simulink model "CMOS_Kernel_Memory_Sync"  (R2023b)
settings: Solver=VariableStepAuto  StartTime=0.0  StopTime=30000000  RelTol=1e-3
values from neighbouring files (symbols this model uses):
  AmountOfPixelsPerScanline = 400    [Kernel_Setup_Script.m]
  AmountOfRamBlocksScanlines = 5    [Kernel_Setup_Script.m]
  AmountOfRamBlocksScanlinesOffset = AmountOfRamBlocksScanlines - 1    (= 4)    [Kernel_Setup_Script.m]
  AmountOfScanlinePixels = 73700    [Kernel_Setup_Script.m]
  AmountOfScanlinePixelsOffset = AmountOfScanlinePixels - 1    (= 73699)    [Kernel_Setup_Script.m]
  AmountOfScanlines = 1100    [Kernel_Setup_Script.m]
  AmountOfScanlinesOffset = AmountOfScanlines - 1    (= 1099)    [Kernel_Setup_Script.m]
  AOPPK_Off = AmountOfPixelsPerScanline - 1    (= 399)    [Kernel_Setup_Script.m]
  AOPPS_Off = AmountOfPixelsPerScanline - 1    (= 399)    [Kernel_Setup_Script.m]
  FramePackOff_0 = FramePackOff_0 - ScanlineFifoCheck    [Kernel_Setup_Script.m]
  FramePackOff_1 = FramePackOff_1 - ScanlineFifoCheck    [Kernel_Setup_Script.m]
  FramePackOff_2 = FramePackOff_2 - ScanlineFifoCheck    [Kernel_Setup_Script.m]
  FramePackOff_3 = FramePackOff_3 - ScanlineFifoCheck    [Kernel_Setup_Script.m]
  FramePackOff_4 = FramePackOff_4 - ScanlineFifoCheck    [Kernel_Setup_Script.m]
  FramePackOff_5 = FramePackOff_5 - ScanlineFifoCheck    [Kernel_Setup_Script.m]
  KernelPackOff_0 = KernelPackOff_0 - KernelBitsPerRow    [Kernel_Setup_Script.m]
  KernelPackOff_1 = KernelPackOff_1 - KernelBitsPerRow    [Kernel_Setup_Script.m]
  KernelPackOff_2 = KernelPackOff_2 - KernelBitsPerRow    [Kernel_Setup_Script.m]
  KernelPackOff_3 = KernelPackOff_3 - KernelBitsPerRow    [Kernel_Setup_Script.m]
  Slice59DownTo48Top = (MsbOffset - (ScanlinePixelBitSizeController*1))    (= 59)    [Kernel_Setup_Script.m]
  Slice71DownTo60Top = (MsbOffset - (ScanlinePixelBitSizeController*0))    (= 71)    [Kernel_Setup_Script.m]
  TotalSectionsForFrames = AmountOfScanlines/AmountOfRamBlocksScanlines    (= 220)    [Kernel_Setup_Script.m]
  UltraRamRows = AmountOfPixelsPerScanline/ScanlineFifoCheck    [Kernel_Setup_Script.m]
  UltraRamRowsCeil = ceil(AmountOfPixelsPerScanline/ScanlineFifoCheck)    [Kernel_Setup_Script.m]
  UltraRamRowsKernel = AmountOfPixelsPerScanline/KernelBitsPerRow    (= 100)    [Kernel_Setup_Script.m]
  UltraRamRowsKernelCeil = ceil(AmountOfPixelsPerScanline/KernelBitsPerRow)    [Kernel_Setup_Script.m]
  UltraRamRowsMemorySectionOffset = UltraRamRowsCeil*AmountOfRamBlocksScanlines    [Kernel_Setup_Script.m]
  UltraRamRowsOffset = UltraRamRowsCeil - 1    [Kernel_Setup_Script.m]
undefined symbols (not defined in the file or in its folder): c, Down, sfvc784, Up, xck26
libraries: hdlBasic x4512, vmcUtilities x1
(part 37 of 39)

== system CMOS_Kernel_Memory_Sync/Memory Handler/Memory Manager/Kernel Memory Subsystem/RAM Selector 2 ==
  Data In : Inport
  RAM Select : Inport  Port=2
  Constant1 : hdlBasic/Constant  const=0  gui_display_data_type=Boolean  arith_type=Boolean  n_bits=1  bin_pt=0  preci_type=Single  exp_width=8  frac_width=24  explicit_period=off  period=1  XmcBlockStatus=1  maskContainerNames=tabcontainer1  block_type=constant  block_config=sysgen:Constant_config
  Delay : hdlBasic/Delay  rst=off  en=off  latency=1  reg_retiming=off  XmcBlockStatus=1  maskContainerNames=group1  block_type=delay  block_config=sysgen:Delay_config
  Line Out RAM {0..4} (5 alike) : hdlBasic/Mux  inputs=2  en=off  latency=1  precision=Full  arith_type=Unsigned  n_bits=16  bin_pt=14  quantization=Truncate  overflow=Wrap  XmcBlockStatus=1  maskContainerNames=tabcontainer1  block_type=mux  block_config=sysgen:Mux_config
  Sel RAM {0..4} (5 alike) : hdlBasic/Relational  mode=a=b  op_type=Bool  en=off  latency=1  XmcBlockStatus=1  maskContainerNames=tabcontainer1  block_type=relational  block_config=sysgen:Relational_config
  Sel Value RAM 0 : hdlBasic/Constant  const=0  gui_display_data_type=Fixed-point  arith_type=Unsigned  n_bits=3  bin_pt=0  preci_type=Single  exp_width=8  frac_width=24  explicit_period=off  period=1  XmcBlockStatus=1  maskContainerNames=tabcontainer1  block_type=constant  block_config=sysgen:Constant_config
  Sel Value RAM 1 : hdlBasic/Constant  const=1  gui_display_data_type=Fixed-point  arith_type=Unsigned  n_bits=3  bin_pt=0  preci_type=Single  exp_width=8  frac_width=24  explicit_period=off  period=1  XmcBlockStatus=1  maskContainerNames=tabcontainer1  block_type=constant  block_config=sysgen:Constant_config
  Sel Value RAM 2 : hdlBasic/Constant  const=2  gui_display_data_type=Fixed-point  arith_type=Unsigned  n_bits=3  bin_pt=0  preci_type=Single  exp_width=8  frac_width=24  explicit_period=off  period=1  XmcBlockStatus=1  maskContainerNames=tabcontainer1  block_type=constant  block_config=sysgen:Constant_config
  Sel Value RAM 3 : hdlBasic/Constant  const=3  gui_display_data_type=Fixed-point  arith_type=Unsigned  n_bits=3  bin_pt=0  preci_type=Single  exp_width=8  frac_width=24  explicit_period=off  period=1  XmcBlockStatus=1  maskContainerNames=tabcontainer1  block_type=constant  block_config=sysgen:Constant_config
  Sel Value RAM 4 : hdlBasic/Constant  const=4  gui_display_data_type=Fixed-point  arith_type=Unsigned  n_bits=3  bin_pt=0  preci_type=Single  exp_width=8  frac_width=24  explicit_period=off  period=1  XmcBlockStatus=1  maskContainerNames=tabcontainer1  block_type=constant  block_config=sysgen:Constant_config
  Out RAM 0 : Outport
  Out RAM 1 : Outport  Port=2
  Out RAM 2 : Outport  Port=3
  Out RAM 3 : Outport  Port=4
  Out RAM 4 : Outport  Port=5
  wires:
  Sel Value RAM 0/1 -> Sel RAM 0/2
  Sel Value RAM 1/1 -> Sel RAM 1/2
  Sel Value RAM 2/1 -> Sel RAM 2/2
  Sel Value RAM 3/1 -> Sel RAM 3/2
  Sel Value RAM 4/1 -> Sel RAM 4/2
  Delay/1 -> Line Out RAM 0/3, Line Out RAM 1/3, Line Out RAM 2/3, Line Out RAM 4/3, Line Out RAM 3/3
  Data In/1 -> Delay/1
  RAM Select/1 -> Sel RAM 4/1, Sel RAM 3/1, Sel RAM 2/1, Sel RAM 1/1, Sel RAM 0/1
  Line Out RAM 0/1 -> Out RAM 0/1
  Line Out RAM 1/1 -> Out RAM 1/1
  Line Out RAM 2/1 -> Out RAM 2/1
  Line Out RAM 3/1 -> Out RAM 3/1
  Line Out RAM 4/1 -> Out RAM 4/1
  Constant1/1 -> Line Out RAM 0/2, Line Out RAM 4/2, Line Out RAM 3/2, Line Out RAM 2/2, Line Out RAM 1/2
  Sel RAM 0/1 -> Line Out RAM 0/1
  Sel RAM 1/1 -> Line Out RAM 1/1
  Sel RAM 2/1 -> Line Out RAM 2/1
  Sel RAM 3/1 -> Line Out RAM 3/1
  Sel RAM 4/1 -> Line Out RAM 4/1

== system CMOS_Kernel_Memory_Sync/Memory Handler/Memory Manager/Scanline Memory Subsystem/RAM Selector 0 ==
  Data In : Inport
  RAM Select : Inport  Port=2
  Constant1 : hdlBasic/Constant  const=0  gui_display_data_type=Fixed-point  arith_type=Unsigned  n_bits=1  bin_pt=0  preci_type=Single  exp_width=8  frac_width=24  explicit_period=off  period=1  XmcBlockStatus=1  maskContainerNames=tabcontainer1  block_type=constant  block_config=sysgen:Constant_config
  Delay : hdlBasic/Delay  rst=off  en=off  latency=1  reg_retiming=off  XmcBlockStatus=1  maskContainerNames=group1  block_type=delay  block_config=sysgen:Delay_config
  Line Out RAM {0..4} (5 alike) : hdlBasic/Mux  inputs=2  en=off  latency=1  precision=Full  arith_type=Unsigned  n_bits=16  bin_pt=14  quantization=Truncate  overflow=Wrap  XmcBlockStatus=1  maskContainerNames=tabcontainer1  block_type=mux  block_config=sysgen:Mux_config
  Sel RAM {0..4} (5 alike) : hdlBasic/Relational  mode=a=b  op_type=Bool  en=off  latency=1  XmcBlockStatus=1  maskContainerNames=tabcontainer1  block_type=relational  block_config=sysgen:Relational_config
  Sel Value RAM 0 : hdlBasic/Constant  const=0  gui_display_data_type=Fixed-point  arith_type=Unsigned  n_bits=3  bin_pt=0  preci_type=Single  exp_width=8  frac_width=24  explicit_period=off  period=1  XmcBlockStatus=1  maskContainerNames=tabcontainer1  block_type=constant  block_config=sysgen:Constant_config
  Sel Value RAM 1 : hdlBasic/Constant  const=1  gui_display_data_type=Fixed-point  arith_type=Unsigned  n_bits=3  bin_pt=0  preci_type=Single  exp_width=8  frac_width=24  explicit_period=off  period=1  XmcBlockStatus=1  maskContainerNames=tabcontainer1  block_type=constant  block_config=sysgen:Constant_config
  Sel Value RAM 2 : hdlBasic/Constant  const=2  gui_display_data_type=Fixed-point  arith_type=Unsigned  n_bits=3  bin_pt=0  preci_type=Single  exp_width=8  frac_width=24  explicit_period=off  period=1  XmcBlockStatus=1  maskContainerNames=tabcontainer1  block_type=constant  block_config=sysgen:Constant_config
  Sel Value RAM 3 : hdlBasic/Constant  const=3  gui_display_data_type=Fixed-point  arith_type=Unsigned  n_bits=3  bin_pt=0  preci_type=Single  exp_width=8  frac_width=24  explicit_period=off  period=1  XmcBlockStatus=1  maskContainerNames=tabcontainer1  block_type=constant  block_config=sysgen:Constant_config
  Sel Value RAM 4 : hdlBasic/Constant  const=4  gui_display_data_type=Fixed-point  arith_type=Unsigned  n_bits=3  bin_pt=0  preci_type=Single  exp_width=8  frac_width=24  explicit_period=off  period=1  XmcBlockStatus=1  maskContainerNames=tabcontainer1  block_type=constant  block_config=sysgen:Constant_config
  Out RAM 0 : Outport
  Out RAM 1 : Outport  Port=2
  Out RAM 2 : Outport  Port=3
  Out RAM 3 : Outport  Port=4
  Out RAM 4 : Outport  Port=5
  wires:
  Sel Value RAM 0/1 -> Sel RAM 0/2
  Sel Value RAM 1/1 -> Sel RAM 1/2
  Sel Value RAM 2/1 -> Sel RAM 2/2
  Sel Value RAM 3/1 -> Sel RAM 3/2
  Sel Value RAM 4/1 -> Sel RAM 4/2
  Delay/1 -> Line Out RAM 0/3, Line Out RAM 1/3, Line Out RAM 2/3, Line Out RAM 4/3, Line Out RAM 3/3
  Data In/1 -> Delay/1
  RAM Select/1 -> Sel RAM 4/1, Sel RAM 3/1, Sel RAM 2/1, Sel RAM 1/1, Sel RAM 0/1
  Line Out RAM 0/1 -> Out RAM 0/1
  Line Out RAM 1/1 -> Out RAM 1/1
  Line Out RAM 2/1 -> Out RAM 2/1
  Line Out RAM 3/1 -> Out RAM 3/1
  Line Out RAM 4/1 -> Out RAM 4/1
  Constant1/1 -> Line Out RAM 0/2, Line Out RAM 4/2, Line Out RAM 3/2, Line Out RAM 2/2, Line Out RAM 1/2
  Sel RAM 0/1 -> Line Out RAM 0/1
  Sel RAM 1/1 -> Line Out RAM 1/1
  Sel RAM 2/1 -> Line Out RAM 2/1
  Sel RAM 3/1 -> Line Out RAM 3/1
  Sel RAM 4/1 -> Line Out RAM 4/1

== system CMOS_Kernel_Memory_Sync/Memory Handler/Memory Manager/Scanline Memory Subsystem/RAM Selector 1 ==
  Data In : Inport
  RAM Select : Inport  Port=2
  Constant1 : hdlBasic/Constant  const=0  gui_display_data_type=Fixed-point  arith_type=Unsigned  n_bits=1  bin_pt=0  preci_type=Single  exp_width=8  frac_width=24  explicit_period=off  period=1  XmcBlockStatus=1  maskContainerNames=tabcontainer1  block_type=constant  block_config=sysgen:Constant_config
  Delay : hdlBasic/Delay  rst=off  en=off  latency=1  reg_retiming=off  XmcBlockStatus=1  maskContainerNames=group1  block_type=delay  block_config=sysgen:Delay_config
  Line Out RAM {0..4} (5 alike) : hdlBasic/Mux  inputs=2  en=off  latency=1  precision=Full  arith_type=Unsigned  n_bits=16  bin_pt=14  quantization=Truncate  overflow=Wrap  XmcBlockStatus=1  maskContainerNames=tabcontainer1  block_type=mux  block_config=sysgen:Mux_config
  Sel RAM {0..4} (5 alike) : hdlBasic/Relational  mode=a=b  op_type=Bool  en=off  latency=1  XmcBlockStatus=1  maskContainerNames=tabcontainer1  block_type=relational  block_config=sysgen:Relational_config
  Sel Value RAM 0 : hdlBasic/Constant  const=0  gui_display_data_type=Fixed-point  arith_type=Unsigned  n_bits=3  bin_pt=0  preci_type=Single  exp_width=8  frac_width=24  explicit_period=off  period=1  XmcBlockStatus=1  maskContainerNames=tabcontainer1  block_type=constant  block_config=sysgen:Constant_config
  Sel Value RAM 1 : hdlBasic/Constant  const=1  gui_display_data_type=Fixed-point  arith_type=Unsigned  n_bits=3  bin_pt=0  preci_type=Single  exp_width=8  frac_width=24  explicit_period=off  period=1  XmcBlockStatus=1  maskContainerNames=tabcontainer1  block_type=constant  block_config=sysgen:Constant_config
  Sel Value RAM 2 : hdlBasic/Constant  const=2  gui_display_data_type=Fixed-point  arith_type=Unsigned  n_bits=3  bin_pt=0  preci_type=Single  exp_width=8  frac_width=24  explicit_period=off  period=1  XmcBlockStatus=1  maskContainerNames=tabcontainer1  block_type=constant  block_config=sysgen:Constant_config
  Sel Value RAM 3 : hdlBasic/Constant  const=3  gui_display_data_type=Fixed-point  arith_type=Unsigned  n_bits=3  bin_pt=0  preci_type=Single  exp_width=8  frac_width=24  explicit_period=off  period=1  XmcBlockStatus=1  maskContainerNames=tabcontainer1  block_type=constant  block_config=sysgen:Constant_config
  Sel Value RAM 4 : hdlBasic/Constant  const=4  gui_display_data_type=Fixed-point  arith_type=Unsigned  n_bits=3  bin_pt=0  preci_type=Single  exp_width=8  frac_width=24  explicit_period=off  period=1  XmcBlockStatus=1  maskContainerNames=tabcontainer1  block_type=constant  block_config=sysgen:Constant_config
  Out RAM 0 : Outport
  Out RAM 1 : Outport  Port=2
  Out RAM 2 : Outport  Port=3
  Out RAM 3 : Outport  Port=4
  Out RAM 4 : Outport  Port=5
  wires:
  Sel Value RAM 0/1 -> Sel RAM 0/2
  Sel Value RAM 1/1 -> Sel RAM 1/2
  Sel Value RAM 2/1 -> Sel RAM 2/2
  Sel Value RAM 3/1 -> Sel RAM 3/2
  Sel Value RAM 4/1 -> Sel RAM 4/2
  Delay/1 -> Line Out RAM 0/3, Line Out RAM 1/3, Line Out RAM 2/3, Line Out RAM 4/3, Line Out RAM 3/3
  Data In/1 -> Delay/1
  RAM Select/1 -> Sel RAM 4/1, Sel RAM 3/1, Sel RAM 2/1, Sel RAM 1/1, Sel RAM 0/1
  Line Out RAM 0/1 -> Out RAM 0/1
  Line Out RAM 1/1 -> Out RAM 1/1
  Line Out RAM 2/1 -> Out RAM 2/1
  Line Out RAM 3/1 -> Out RAM 3/1
  Line Out RAM 4/1 -> Out RAM 4/1
  Constant1/1 -> Line Out RAM 0/2, Line Out RAM 4/2, Line Out RAM 3/2, Line Out RAM 2/2, Line Out RAM 1/2
  Sel RAM 0/1 -> Line Out RAM 0/1
  Sel RAM 1/1 -> Line Out RAM 1/1
  Sel RAM 2/1 -> Line Out RAM 2/1
  Sel RAM 3/1 -> Line Out RAM 3/1
  Sel RAM 4/1 -> Line Out RAM 4/1

== system CMOS_Kernel_Memory_Sync/Memory Handler/Memory Manager/Scanline Memory Subsystem/RAM Selector 2 ==
  Data In : Inport
  RAM Select : Inport  Port=2
  Constant1 : hdlBasic/Constant  const=0  gui_display_data_type=Boolean  arith_type=Boolean  n_bits=1  bin_pt=0  preci_type=Single  exp_width=8  frac_width=24  explicit_period=off  period=1  XmcBlockStatus=1  maskContainerNames=tabcontainer1  block_type=constant  block_config=sysgen:Constant_config
  Delay : hdlBasic/Delay  rst=off  en=off  latency=1  reg_retiming=off  XmcBlockStatus=1  maskContainerNames=group1  block_type=delay  block_config=sysgen:Delay_config
  Line Out RAM {0..4} (5 alike) : hdlBasic/Mux  inputs=2  en=off  latency=1  precision=Full  arith_type=Unsigned  n_bits=16  bin_pt=14  quantization=Truncate  overflow=Wrap  XmcBlockStatus=1  maskContainerNames=tabcontainer1  block_type=mux  block_config=sysgen:Mux_config
  Sel RAM {0..4} (5 alike) : hdlBasic/Relational  mode=a=b  op_type=Bool  en=off  latency=1  XmcBlockStatus=1  maskContainerNames=tabcontainer1  block_type=relational  block_config=sysgen:Relational_config
  Sel Value RAM 0 : hdlBasic/Constant  const=0  gui_display_data_type=Fixed-point  arith_type=Unsigned  n_bits=3  bin_pt=0  preci_type=Single  exp_width=8  frac_width=24  explicit_period=off  period=1  XmcBlockStatus=1  maskContainerNames=tabcontainer1  block_type=constant  block_config=sysgen:Constant_config
  Sel Value RAM 1 : hdlBasic/Constant  const=1  gui_display_data_type=Fixed-point  arith_type=Unsigned  n_bits=3  bin_pt=0  preci_type=Single  exp_width=8  frac_width=24  explicit_period=off  period=1  XmcBlockStatus=1  maskContainerNames=tabcontainer1  block_type=constant  block_config=sysgen:Constant_config
  Sel Value RAM 2 : hdlBasic/Constant  const=2  gui_display_data_type=Fixed-point  arith_type=Unsigned  n_bits=3  bin_pt=0  preci_type=Single  exp_width=8  frac_width=24  explicit_period=off  period=1  XmcBlockStatus=1  maskContainerNames=tabcontainer1  block_type=constant  block_config=sysgen:Constant_config
  Sel Value RAM 3 : hdlBasic/Constant  const=3  gui_display_data_type=Fixed-point  arith_type=Unsigned  n_bits=3  bin_pt=0  preci_type=Single  exp_width=8  frac_width=24  explicit_period=off  period=1  XmcBlockStatus=1  maskContainerNames=tabcontainer1  block_type=constant  block_config=sysgen:Constant_config
  Sel Value RAM 4 : hdlBasic/Constant  const=4  gui_display_data_type=Fixed-point  arith_type=Unsigned  n_bits=3  bin_pt=0  preci_type=Single  exp_width=8  frac_width=24  explicit_period=off  period=1  XmcBlockStatus=1  maskContainerNames=tabcontainer1  block_type=constant  block_config=sysgen:Constant_config
  Out RAM 0 : Outport
  Out RAM 1 : Outport  Port=2
  Out RAM 2 : Outport  Port=3
  Out RAM 3 : Outport  Port=4
  Out RAM 4 : Outport  Port=5
  wires:
  Sel Value RAM 0/1 -> Sel RAM 0/2
  Sel Value RAM 1/1 -> Sel RAM 1/2
  Sel Value RAM 2/1 -> Sel RAM 2/2
  Sel Value RAM 3/1 -> Sel RAM 3/2
  Sel Value RAM 4/1 -> Sel RAM 4/2
  Delay/1 -> Line Out RAM 0/3, Line Out RAM 1/3, Line Out RAM 2/3, Line Out RAM 4/3, Line Out RAM 3/3
  Data In/1 -> Delay/1
  RAM Select/1 -> Sel RAM 4/1, Sel RAM 3/1, Sel RAM 2/1, Sel RAM 1/1, Sel RAM 0/1
  Line Out RAM 0/1 -> Out RAM 0/1
  Line Out RAM 1/1 -> Out RAM 1/1
  Line Out RAM 2/1 -> Out RAM 2/1
  Line Out RAM 3/1 -> Out RAM 3/1
  Line Out RAM 4/1 -> Out RAM 4/1
  Constant1/1 -> Line Out RAM 0/2, Line Out RAM 4/2, Line Out RAM 3/2, Line Out RAM 2/2, Line Out RAM 1/2
  Sel RAM 0/1 -> Line Out RAM 0/1
  Sel RAM 1/1 -> Line Out RAM 1/1
  Sel RAM 2/1 -> Line Out RAM 2/1
  Sel RAM 3/1 -> Line Out RAM 3/1
  Sel RAM 4/1 -> Line Out RAM 4/1

== system CMOS_Kernel_Memory_Sync/Memory Handler/Data Slicer/Frame RAM Slicer/72 Bit Unpacker RAM 0/Unpack 72 Bit FIFO 0 ==
  72 Bit Input : Inport
  Slice 11 Down To 0 : hdlBasic/Slice  nbits=ScanlinePixelBitSizeController  boolean_output=off  mode=Upper Bit Location + Width  bit1=Slice11DownTo0Top  base1=LSB of Input  bit0=0  base0=Binary Point of Input  XmcBlockStatus=1  maskContainerNames=group1  block_type=slice  block_config=sysgen:Slice_config
  Slice 23 Down To 12 : hdlBasic/Slice  nbits=ScanlinePixelBitSizeController  boolean_output=off  mode=Upper Bit Location + Width  bit1=Slice23DownTo12Top  base1=LSB of Input  bit0=12  base0=Binary Point of Input  XmcBlockStatus=1  maskContainerNames=group1  block_type=slice  block_config=sysgen:Slice_config
  Slice 35 Down To 24 : hdlBasic/Slice  nbits=ScanlinePixelBitSizeController  boolean_output=off  mode=Upper Bit Location + Width  bit1=Slice35DownTo24Top  base1=LSB of Input  bit0=24  base0=Binary Point of Input  XmcBlockStatus=1  maskContainerNames=group1  block_type=slice  block_config=sysgen:Slice_config
  Slice 47 Down To 36 : hdlBasic/Slice  nbits=ScanlinePixelBitSizeController  boolean_output=off  mode=Upper Bit Location + Width  bit1=Slice47DownTo36Top  base1=LSB of Input  bit0=36  base0=Binary Point of Input  XmcBlockStatus=1  maskContainerNames=group1  block_type=slice  block_config=sysgen:Slice_config
  Slice 59 Down To 48 : hdlBasic/Slice  nbits=ScanlinePixelBitSizeController  boolean_output=off  mode=Upper Bit Location + Width  bit1=Slice59DownTo48Top  base1=LSB of Input  bit0=Slice59DownTo48Top - 11  base0=LSB of Input  XmcBlockStatus=1  maskContainerNames=group1  block_type=slice  block_config=sysgen:Slice_config
  Slice 71 Down To 60 : hdlBasic/Slice  nbits=ScanlinePixelBitSizeController  boolean_output=off  mode=Upper Bit Location + Width  bit1=Slice71DownTo60Top  base1=LSB of Input  bit0=Slice71DownTo60Top - 12  base0=LSB of Input  XmcBlockStatus=1  maskContainerNames=group1  block_type=slice  block_config=sysgen:Slice_config
  71 Downto 60 : Outport
  59 Downto 48 : Outport  Port=2
  47 Downto 36 : Outport  Port=3
  35 Downto 24 : Outport  Port=4
  23 Downto 12 : Outport  Port=5
  11 Downto 0 : Outport  Port=6
  wires:
  72 Bit Input/1 -> Slice 11 Down To 0/1, Slice 23 Down To 12/1, Slice 35 Down To 24/1, Slice 47 Down To 36/1, Slice 59 Down To 48/1, Slice 71 Down To 60/1
  Slice 23 Down To 12/1 -> 23 Downto 12/1
  Slice 47 Down To 36/1 -> 47 Downto 36/1
  Slice 59 Down To 48/1 -> 59 Downto 48/1
  Slice 35 Down To 24/1 -> 35 Downto 24/1
  Slice 71 Down To 60/1 -> 71 Downto 60/1
  Slice 11 Down To 0/1 -> 11 Downto 0/1

== system CMOS_Kernel_Memory_Sync/Memory Handler/Data Slicer/Frame RAM Slicer/72 Bit Unpacker RAM 0/Unpack 72 Bit FIFO 1 ==
  72 Bit Input : Inport
  Slice 11 Down To 0 : hdlBasic/Slice  nbits=ScanlinePixelBitSizeController  boolean_output=off  mode=Upper Bit Location + Width  bit1=Slice11DownTo0Top  base1=LSB of Input  bit0=0  base0=Binary Point of Input  XmcBlockStatus=1  maskContainerNames=group1  block_type=slice  block_config=sysgen:Slice_config
  Slice 23 Down To 12 : hdlBasic/Slice  nbits=ScanlinePixelBitSizeController  boolean_output=off  mode=Upper Bit Location + Width  bit1=Slice23DownTo12Top  base1=LSB of Input  bit0=12  base0=Binary Point of Input  XmcBlockStatus=1  maskContainerNames=group1  block_type=slice  block_config=sysgen:Slice_config
  Slice 35 Down To 24 : hdlBasic/Slice  nbits=ScanlinePixelBitSizeController  boolean_output=off  mode=Upper Bit Location + Width  bit1=Slice35DownTo24Top  base1=LSB of Input  bit0=24  base0=Binary Point of Input  XmcBlockStatus=1  maskContainerNames=group1  block_type=slice  block_config=sysgen:Slice_config
  Slice 47 Down To 36 : hdlBasic/Slice  nbits=ScanlinePixelBitSizeController  boolean_output=off  mode=Upper Bit Location + Width  bit1=Slice47DownTo36Top  base1=LSB of Input  bit0=36  base0=Binary Point of Input  XmcBlockStatus=1  maskContainerNames=group1  block_type=slice  block_config=sysgen:Slice_config
  Slice 59 Down To 48 : hdlBasic/Slice  nbits=ScanlinePixelBitSizeController  boolean_output=off  mode=Upper Bit Location + Width  bit1=Slice59DownTo48Top  base1=LSB of Input  bit0=48  base0=Binary Point of Input  XmcBlockStatus=1  maskContainerNames=group1  block_type=slice  block_config=sysgen:Slice_config
  Slice 71 Down To 60 : hdlBasic/Slice  nbits=ScanlinePixelBitSizeController  boolean_output=off  mode=Upper Bit Location + Width  bit1=Slice71DownTo60Top  base1=LSB of Input  bit0=Slice71DownTo60Botttom  base0=LSB of Input  XmcBlockStatus=1  maskContainerNames=group1  block_type=slice  block_config=sysgen:Slice_config
  71 Downto 60 : Outport
  59 Downto 48 : Outport  Port=2
  47 Downto 36 : Outport  Port=3
  35 Downto 24 : Outport  Port=4
  23 Downto 12 : Outport  Port=5
  11 Downto 0 : Outport  Port=6
  wires:
  72 Bit Input/1 -> Slice 11 Down To 0/1, Slice 23 Down To 12/1, Slice 35 Down To 24/1, Slice 47 Down To 36/1, Slice 59 Down To 48/1, Slice 71 Down To 60/1
  Slice 23 Down To 12/1 -> 23 Downto 12/1
  Slice 47 Down To 36/1 -> 47 Downto 36/1
  Slice 59 Down To 48/1 -> 59 Downto 48/1
  Slice 35 Down To 24/1 -> 35 Downto 24/1
  Slice 71 Down To 60/1 -> 71 Downto 60/1
  Slice 11 Down To 0/1 -> 11 Downto 0/1

== system CMOS_Kernel_Memory_Sync/Memory Handler/Data Slicer/Frame RAM Slicer/72 Bit Unpacker RAM 1/Unpack 72 Bit FIFO 0 ==
  72 Bit Input : Inport
  Slice 11 Down To 0 : hdlBasic/Slice  nbits=ScanlinePixelBitSizeController  boolean_output=off  mode=Upper Bit Location + Width  bit1=Slice11DownTo0Top  base1=LSB of Input  bit0=0  base0=Binary Point of Input  XmcBlockStatus=1  maskContainerNames=group1  block_type=slice  block_config=sysgen:Slice_config
  Slice 23 Down To 12 : hdlBasic/Slice  nbits=ScanlinePixelBitSizeController  boolean_output=off  mode=Upper Bit Location + Width  bit1=Slice23DownTo12Top  base1=LSB of Input  bit0=12  base0=Binary Point of Input  XmcBlockStatus=1  maskContainerNames=group1  block_type=slice  block_config=sysgen:Slice_config
  Slice 35 Down To 24 : hdlBasic/Slice  nbits=ScanlinePixelBitSizeController  boolean_output=off  mode=Upper Bit Location + Width  bit1=Slice35DownTo24Top  base1=LSB of Input  bit0=24  base0=Binary Point of Input  XmcBlockStatus=1  maskContainerNames=group1  block_type=slice  block_config=sysgen:Slice_config
  Slice 47 Down To 36 : hdlBasic/Slice  nbits=ScanlinePixelBitSizeController  boolean_output=off  mode=Upper Bit Location + Width  bit1=Slice47DownTo36Top  base1=LSB of Input  bit0=36  base0=Binary Point of Input  XmcBlockStatus=1  maskContainerNames=group1  block_type=slice  block_config=sysgen:Slice_config
  Slice 59 Down To 48 : hdlBasic/Slice  nbits=ScanlinePixelBitSizeController  boolean_output=off  mode=Upper Bit Location + Width  bit1=Slice59DownTo48Top  base1=LSB of Input  bit0=Slice59DownTo48Top - 11  base0=LSB of Input  XmcBlockStatus=1  maskContainerNames=group1  block_type=slice  block_config=sysgen:Slice_config
  Slice 71 Down To 60 : hdlBasic/Slice  nbits=ScanlinePixelBitSizeController  boolean_output=off  mode=Upper Bit Location + Width  bit1=Slice71DownTo60Top  base1=LSB of Input  bit0=Slice71DownTo60Top - 12  base0=LSB of Input  XmcBlockStatus=1  maskContainerNames=group1  block_type=slice  block_config=sysgen:Slice_config
  71 Downto 60 : Outport
  59 Downto 48 : Outport  Port=2
  47 Downto 36 : Outport  Port=3
  35 Downto 24 : Outport  Port=4
  23 Downto 12 : Outport  Port=5
  11 Downto 0 : Outport  Port=6
  wires:
  72 Bit Input/1 -> Slice 11 Down To 0/1, Slice 23 Down To 12/1, Slice 35 Down To 24/1, Slice 47 Down To 36/1, Slice 59 Down To 48/1, Slice 71 Down To 60/1
  Slice 23 Down To 12/1 -> 23 Downto 12/1
  Slice 47 Down To 36/1 -> 47 Downto 36/1
  Slice 59 Down To 48/1 -> 59 Downto 48/1
  Slice 35 Down To 24/1 -> 35 Downto 24/1
  Slice 71 Down To 60/1 -> 71 Downto 60/1
  Slice 11 Down To 0/1 -> 11 Downto 0/1

== system CMOS_Kernel_Memory_Sync/Memory Handler/Data Slicer/Frame RAM Slicer/72 Bit Unpacker RAM 1/Unpack 72 Bit FIFO 1 ==
  72 Bit Input : Inport
  Slice 11 Down To 0 : hdlBasic/Slice  nbits=ScanlinePixelBitSizeController  boolean_output=off  mode=Upper Bit Location + Width  bit1=Slice11DownTo0Top  base1=LSB of Input  bit0=0  base0=Binary Point of Input  XmcBlockStatus=1  maskContainerNames=group1  block_type=slice  block_config=sysgen:Slice_config
  Slice 23 Down To 12 : hdlBasic/Slice  nbits=ScanlinePixelBitSizeController  boolean_output=off  mode=Upper Bit Location + Width  bit1=Slice23DownTo12Top  base1=LSB of Input  bit0=12  base0=Binary Point of Input  XmcBlockStatus=1  maskContainerNames=group1  block_type=slice  block_config=sysgen:Slice_config
  Slice 35 Down To 24 : hdlBasic/Slice  nbits=ScanlinePixelBitSizeController  boolean_output=off  mode=Upper Bit Location + Width  bit1=Slice35DownTo24Top  base1=LSB of Input  bit0=24  base0=Binary Point of Input  XmcBlockStatus=1  maskContainerNames=group1  block_type=slice  block_config=sysgen:Slice_config
  Slice 47 Down To 36 : hdlBasic/Slice  nbits=ScanlinePixelBitSizeController  boolean_output=off  mode=Upper Bit Location + Width  bit1=Slice47DownTo36Top  base1=LSB of Input  bit0=36  base0=Binary Point of Input  XmcBlockStatus=1  maskContainerNames=group1  block_type=slice  block_config=sysgen:Slice_config
  Slice 59 Down To 48 : hdlBasic/Slice  nbits=ScanlinePixelBitSizeController  boolean_output=off  mode=Upper Bit Location + Width  bit1=Slice59DownTo48Top  base1=LSB of Input  bit0=48  base0=Binary Point of Input  XmcBlockStatus=1  maskContainerNames=group1  block_type=slice  block_config=sysgen:Slice_config
  Slice 71 Down To 60 : hdlBasic/Slice  nbits=ScanlinePixelBitSizeController  boolean_output=off  mode=Upper Bit Location + Width  bit1=Slice71DownTo60Top  base1=LSB of Input  bit0=Slice71DownTo60Botttom  base0=LSB of Input  XmcBlockStatus=1  maskContainerNames=group1  block_type=slice  block_config=sysgen:Slice_config
  71 Downto 60 : Outport
  59 Downto 48 : Outport  Port=2
  47 Downto 36 : Outport  Port=3
  35 Downto 24 : Outport  Port=4
  23 Downto 12 : Outport  Port=5
  11 Downto 0 : Outport  Port=6
  wires:
  72 Bit Input/1 -> Slice 11 Down To 0/1, Slice 23 Down To 12/1, Slice 35 Down To 24/1, Slice 47 Down To 36/1, Slice 59 Down To 48/1, Slice 71 Down To 60/1
  Slice 23 Down To 12/1 -> 23 Downto 12/1
  Slice 47 Down To 36/1 -> 47 Downto 36/1
  Slice 59 Down To 48/1 -> 59 Downto 48/1
  Slice 35 Down To 24/1 -> 35 Downto 24/1
  Slice 71 Down To 60/1 -> 71 Downto 60/1
  Slice 11 Down To 0/1 -> 11 Downto 0/1

== system CMOS_Kernel_Memory_Sync/Memory Handler/Data Slicer/Frame RAM Slicer/72 Bit Unpacker RAM 2/Unpack 72 Bit FIFO 0 ==
  72 Bit Input : Inport
  Slice 11 Down To 0 : hdlBasic/Slice  nbits=ScanlinePixelBitSizeController  boolean_output=off  mode=Upper Bit Location + Width  bit1=Slice11DownTo0Top  base1=LSB of Input  bit0=0  base0=Binary Point of Input  XmcBlockStatus=1  maskContainerNames=group1  block_type=slice  block_config=sysgen:Slice_config
  Slice 23 Down To 12 : hdlBasic/Slice  nbits=ScanlinePixelBitSizeController  boolean_output=off  mode=Upper Bit Location + Width  bit1=Slice23DownTo12Top  base1=LSB of Input  bit0=12  base0=Binary Point of Input  XmcBlockStatus=1  maskContainerNames=group1  block_type=slice  block_config=sysgen:Slice_config
  Slice 35 Down To 24 : hdlBasic/Slice  nbits=ScanlinePixelBitSizeController  boolean_output=off  mode=Upper Bit Location + Width  bit1=Slice35DownTo24Top  base1=LSB of Input  bit0=24  base0=Binary Point of Input  XmcBlockStatus=1  maskContainerNames=group1  block_type=slice  block_config=sysgen:Slice_config
  Slice 47 Down To 36 : hdlBasic/Slice  nbits=ScanlinePixelBitSizeController  boolean_output=off  mode=Upper Bit Location + Width  bit1=Slice47DownTo36Top  base1=LSB of Input  bit0=36  base0=Binary Point of Input  XmcBlockStatus=1  maskContainerNames=group1  block_type=slice  block_config=sysgen:Slice_config
  Slice 59 Down To 48 : hdlBasic/Slice  nbits=ScanlinePixelBitSizeController  boolean_output=off  mode=Upper Bit Location + Width  bit1=Slice59DownTo48Top  base1=LSB of Input  bit0=Slice59DownTo48Top - 11  base0=LSB of Input  XmcBlockStatus=1  maskContainerNames=group1  block_type=slice  block_config=sysgen:Slice_config
  Slice 71 Down To 60 : hdlBasic/Slice  nbits=ScanlinePixelBitSizeController  boolean_output=off  mode=Upper Bit Location + Width  bit1=Slice71DownTo60Top  base1=LSB of Input  bit0=Slice71DownTo60Top - 12  base0=LSB of Input  XmcBlockStatus=1  maskContainerNames=group1  block_type=slice  block_config=sysgen:Slice_config
  71 Downto 60 : Outport
  59 Downto 48 : Outport  Port=2
  47 Downto 36 : Outport  Port=3
  35 Downto 24 : Outport  Port=4
  23 Downto 12 : Outport  Port=5
  11 Downto 0 : Outport  Port=6
  wires:
  72 Bit Input/1 -> Slice 11 Down To 0/1, Slice 23 Down To 12/1, Slice 35 Down To 24/1, Slice 47 Down To 36/1, Slice 59 Down To 48/1, Slice 71 Down To 60/1
  Slice 23 Down To 12/1 -> 23 Downto 12/1
  Slice 47 Down To 36/1 -> 47 Downto 36/1
  Slice 59 Down To 48/1 -> 59 Downto 48/1
  Slice 35 Down To 24/1 -> 35 Downto 24/1
  Slice 71 Down To 60/1 -> 71 Downto 60/1
  Slice 11 Down To 0/1 -> 11 Downto 0/1

== system CMOS_Kernel_Memory_Sync/Memory Handler/Data Slicer/Frame RAM Slicer/72 Bit Unpacker RAM 2/Unpack 72 Bit FIFO 1 ==
  72 Bit Input : Inport
  Slice 11 Down To 0 : hdlBasic/Slice  nbits=ScanlinePixelBitSizeController  boolean_output=off  mode=Upper Bit Location + Width  bit1=Slice11DownTo0Top  base1=LSB of Input  bit0=0  base0=Binary Point of Input  XmcBlockStatus=1  maskContainerNames=group1  block_type=slice  block_config=sysgen:Slice_config
  Slice 23 Down To 12 : hdlBasic/Slice  nbits=ScanlinePixelBitSizeController  boolean_output=off  mode=Upper Bit Location + Width  bit1=Slice23DownTo12Top  base1=LSB of Input  bit0=12  base0=Binary Point of Input  XmcBlockStatus=1  maskContainerNames=group1  block_type=slice  block_config=sysgen:Slice_config
  Slice 35 Down To 24 : hdlBasic/Slice  nbits=ScanlinePixelBitSizeController  boolean_output=off  mode=Upper Bit Location + Width  bit1=Slice35DownTo24Top  base1=LSB of Input  bit0=24  base0=Binary Point of Input  XmcBlockStatus=1  maskContainerNames=group1  block_type=slice  block_config=sysgen:Slice_config
  Slice 47 Down To 36 : hdlBasic/Slice  nbits=ScanlinePixelBitSizeController  boolean_output=off  mode=Upper Bit Location + Width  bit1=Slice47DownTo36Top  base1=LSB of Input  bit0=36  base0=Binary Point of Input  XmcBlockStatus=1  maskContainerNames=group1  block_type=slice  block_config=sysgen:Slice_config
  Slice 59 Down To 48 : hdlBasic/Slice  nbits=ScanlinePixelBitSizeController  boolean_output=off  mode=Upper Bit Location + Width  bit1=Slice59DownTo48Top  base1=LSB of Input  bit0=48  base0=Binary Point of Input  XmcBlockStatus=1  maskContainerNames=group1  block_type=slice  block_config=sysgen:Slice_config
  Slice 71 Down To 60 : hdlBasic/Slice  nbits=ScanlinePixelBitSizeController  boolean_output=off  mode=Upper Bit Location + Width  bit1=Slice71DownTo60Top  base1=LSB of Input  bit0=Slice71DownTo60Botttom  base0=LSB of Input  XmcBlockStatus=1  maskContainerNames=group1  block_type=slice  block_config=sysgen:Slice_config
  71 Downto 60 : Outport
  59 Downto 48 : Outport  Port=2
  47 Downto 36 : Outport  Port=3
  35 Downto 24 : Outport  Port=4
  23 Downto 12 : Outport  Port=5
  11 Downto 0 : Outport  Port=6
  wires:
  72 Bit Input/1 -> Slice 11 Down To 0/1, Slice 23 Down To 12/1, Slice 35 Down To 24/1, Slice 47 Down To 36/1, Slice 59 Down To 48/1, Slice 71 Down To 60/1
  Slice 23 Down To 12/1 -> 23 Downto 12/1
  Slice 47 Down To 36/1 -> 47 Downto 36/1
  Slice 59 Down To 48/1 -> 59 Downto 48/1
  Slice 35 Down To 24/1 -> 35 Downto 24/1
  Slice 71 Down To 60/1 -> 71 Downto 60/1
  Slice 11 Down To 0/1 -> 11 Downto 0/1

== system CMOS_Kernel_Memory_Sync/Memory Handler/Data Slicer/Frame RAM Slicer/72 Bit Unpacker RAM 3/Unpack 72 Bit FIFO 0 ==
  72 Bit Input : Inport
  Slice 11 Down To 0 : hdlBasic/Slice  nbits=ScanlinePixelBitSizeController  boolean_output=off  mode=Upper Bit Location + Width  bit1=Slice11DownTo0Top  base1=LSB of Input  bit0=0  base0=Binary Point of Input  XmcBlockStatus=1  maskContainerNames=group1  block_type=slice  block_config=sysgen:Slice_config
  Slice 23 Down To 12 : hdlBasic/Slice  nbits=ScanlinePixelBitSizeController  boolean_output=off  mode=Upper Bit Location + Width  bit1=Slice23DownTo12Top  base1=LSB of Input  bit0=12  base0=Binary Point of Input  XmcBlockStatus=1  maskContainerNames=group1  block_type=slice  block_config=sysgen:Slice_config
  Slice 35 Down To 24 : hdlBasic/Slice  nbits=ScanlinePixelBitSizeController  boolean_output=off  mode=Upper Bit Location + Width  bit1=Slice35DownTo24Top  base1=LSB of Input  bit0=24  base0=Binary Point of Input  XmcBlockStatus=1  maskContainerNames=group1  block_type=slice  block_config=sysgen:Slice_config
  Slice 47 Down To 36 : hdlBasic/Slice  nbits=ScanlinePixelBitSizeController  boolean_output=off  mode=Upper Bit Location + Width  bit1=Slice47DownTo36Top  base1=LSB of Input  bit0=36  base0=Binary Point of Input  XmcBlockStatus=1  maskContainerNames=group1  block_type=slice  block_config=sysgen:Slice_config
  Slice 59 Down To 48 : hdlBasic/Slice  nbits=ScanlinePixelBitSizeController  boolean_output=off  mode=Upper Bit Location + Width  bit1=Slice59DownTo48Top  base1=LSB of Input  bit0=Slice59DownTo48Top - 11  base0=LSB of Input  XmcBlockStatus=1  maskContainerNames=group1  block_type=slice  block_config=sysgen:Slice_config
  Slice 71 Down To 60 : hdlBasic/Slice  nbits=ScanlinePixelBitSizeController  boolean_output=off  mode=Upper Bit Location + Width  bit1=Slice71DownTo60Top  base1=LSB of Input  bit0=Slice71DownTo60Top - 12  base0=LSB of Input  XmcBlockStatus=1  maskContainerNames=group1  block_type=slice  block_config=sysgen:Slice_config
  71 Downto 60 : Outport
  59 Downto 48 : Outport  Port=2
  47 Downto 36 : Outport  Port=3
  35 Downto 24 : Outport  Port=4
  23 Downto 12 : Outport  Port=5
  11 Downto 0 : Outport  Port=6
  wires:
  72 Bit Input/1 -> Slice 11 Down To 0/1, Slice 23 Down To 12/1, Slice 35 Down To 24/1, Slice 47 Down To 36/1, Slice 59 Down To 48/1, Slice 71 Down To 60/1
  Slice 23 Down To 12/1 -> 23 Downto 12/1
  Slice 47 Down To 36/1 -> 47 Downto 36/1
  Slice 59 Down To 48/1 -> 59 Downto 48/1
  Slice 35 Down To 24/1 -> 35 Downto 24/1
  Slice 71 Down To 60/1 -> 71 Downto 60/1
  Slice 11 Down To 0/1 -> 11 Downto 0/1

== system CMOS_Kernel_Memory_Sync/Memory Handler/Data Slicer/Frame RAM Slicer/72 Bit Unpacker RAM 3/Unpack 72 Bit FIFO 1 ==
  72 Bit Input : Inport
  Slice 11 Down To 0 : hdlBasic/Slice  nbits=ScanlinePixelBitSizeController  boolean_output=off  mode=Upper Bit Location + Width  bit1=Slice11DownTo0Top  base1=LSB of Input  bit0=0  base0=Binary Point of Input  XmcBlockStatus=1  maskContainerNames=group1  block_type=slice  block_config=sysgen:Slice_config
  Slice 23 Down To 12 : hdlBasic/Slice  nbits=ScanlinePixelBitSizeController  boolean_output=off  mode=Upper Bit Location + Width  bit1=Slice23DownTo12Top  base1=LSB of Input  bit0=12  base0=Binary Point of Input  XmcBlockStatus=1  maskContainerNames=group1  block_type=slice  block_config=sysgen:Slice_config
  Slice 35 Down To 24 : hdlBasic/Slice  nbits=ScanlinePixelBitSizeController  boolean_output=off  mode=Upper Bit Location + Width  bit1=Slice35DownTo24Top  base1=LSB of Input  bit0=24  base0=Binary Point of Input  XmcBlockStatus=1  maskContainerNames=group1  block_type=slice  block_config=sysgen:Slice_config
  Slice 47 Down To 36 : hdlBasic/Slice  nbits=ScanlinePixelBitSizeController  boolean_output=off  mode=Upper Bit Location + Width  bit1=Slice47DownTo36Top  base1=LSB of Input  bit0=36  base0=Binary Point of Input  XmcBlockStatus=1  maskContainerNames=group1  block_type=slice  block_config=sysgen:Slice_config
  Slice 59 Down To 48 : hdlBasic/Slice  nbits=ScanlinePixelBitSizeController  boolean_output=off  mode=Upper Bit Location + Width  bit1=Slice59DownTo48Top  base1=LSB of Input  bit0=48  base0=Binary Point of Input  XmcBlockStatus=1  maskContainerNames=group1  block_type=slice  block_config=sysgen:Slice_config
  Slice 71 Down To 60 : hdlBasic/Slice  nbits=ScanlinePixelBitSizeController  boolean_output=off  mode=Upper Bit Location + Width  bit1=Slice71DownTo60Top  base1=LSB of Input  bit0=Slice71DownTo60Botttom  base0=LSB of Input  XmcBlockStatus=1  maskContainerNames=group1  block_type=slice  block_config=sysgen:Slice_config
  71 Downto 60 : Outport
  59 Downto 48 : Outport  Port=2
  47 Downto 36 : Outport  Port=3
  35 Downto 24 : Outport  Port=4
  23 Downto 12 : Outport  Port=5
  11 Downto 0 : Outport  Port=6
  wires:
  72 Bit Input/1 -> Slice 11 Down To 0/1, Slice 23 Down To 12/1, Slice 35 Down To 24/1, Slice 47 Down To 36/1, Slice 59 Down To 48/1, Slice 71 Down To 60/1
  Slice 23 Down To 12/1 -> 23 Downto 12/1
  Slice 47 Down To 36/1 -> 47 Downto 36/1
  Slice 59 Down To 48/1 -> 59 Downto 48/1
  Slice 35 Down To 24/1 -> 35 Downto 24/1
  Slice 71 Down To 60/1 -> 71 Downto 60/1
  Slice 11 Down To 0/1 -> 11 Downto 0/1

== system CMOS_Kernel_Memory_Sync/Memory Handler/Data Slicer/Frame RAM Slicer/72 Bit Unpacker RAM 4/Unpack 72 Bit FIFO 0 ==
  72 Bit Input : Inport
  Slice 11 Down To 0 : hdlBasic/Slice  nbits=ScanlinePixelBitSizeController  boolean_output=off  mode=Upper Bit Location + Width  bit1=Slice11DownTo0Top  base1=LSB of Input  bit0=0  base0=Binary Point of Input  XmcBlockStatus=1  maskContainerNames=group1  block_type=slice  block_config=sysgen:Slice_config
  Slice 23 Down To 12 : hdlBasic/Slice  nbits=ScanlinePixelBitSizeController  boolean_output=off  mode=Upper Bit Location + Width  bit1=Slice23DownTo12Top  base1=LSB of Input  bit0=12  base0=Binary Point of Input  XmcBlockStatus=1  maskContainerNames=group1  block_type=slice  block_config=sysgen:Slice_config
  Slice 35 Down To 24 : hdlBasic/Slice  nbits=ScanlinePixelBitSizeController  boolean_output=off  mode=Upper Bit Location + Width  bit1=Slice35DownTo24Top  base1=LSB of Input  bit0=24  base0=Binary Point of Input  XmcBlockStatus=1  maskContainerNames=group1  block_type=slice  block_config=sysgen:Slice_config
  Slice 47 Down To 36 : hdlBasic/Slice  nbits=ScanlinePixelBitSizeController  boolean_output=off  mode=Upper Bit Location + Width  bit1=Slice47DownTo36Top  base1=LSB of Input  bit0=36  base0=Binary Point of Input  XmcBlockStatus=1  maskContainerNames=group1  block_type=slice  block_config=sysgen:Slice_config
  Slice 59 Down To 48 : hdlBasic/Slice  nbits=ScanlinePixelBitSizeController  boolean_output=off  mode=Upper Bit Location + Width  bit1=Slice59DownTo48Top  base1=LSB of Input  bit0=Slice59DownTo48Top - 11  base0=LSB of Input  XmcBlockStatus=1  maskContainerNames=group1  block_type=slice  block_config=sysgen:Slice_config
  Slice 71 Down To 60 : hdlBasic/Slice  nbits=ScanlinePixelBitSizeController  boolean_output=off  mode=Upper Bit Location + Width  bit1=Slice71DownTo60Top  base1=LSB of Input  bit0=Slice71DownTo60Top - 12  base0=LSB of Input  XmcBlockStatus=1  maskContainerNames=group1  block_type=slice  block_config=sysgen:Slice_config
  71 Downto 60 : Outport
  59 Downto 48 : Outport  Port=2
  47 Downto 36 : Outport  Port=3
  35 Downto 24 : Outport  Port=4
  23 Downto 12 : Outport  Port=5
  11 Downto 0 : Outport  Port=6
  wires:
  72 Bit Input/1 -> Slice 11 Down To 0/1, Slice 23 Down To 12/1, Slice 35 Down To 24/1, Slice 47 Down To 36/1, Slice 59 Down To 48/1, Slice 71 Down To 60/1
  Slice 23 Down To 12/1 -> 23 Downto 12/1
  Slice 47 Down To 36/1 -> 47 Downto 36/1
  Slice 59 Down To 48/1 -> 59 Downto 48/1
  Slice 35 Down To 24/1 -> 35 Downto 24/1
  Slice 71 Down To 60/1 -> 71 Downto 60/1
  Slice 11 Down To 0/1 -> 11 Downto 0/1

== system CMOS_Kernel_Memory_Sync/Memory Handler/Data Slicer/Frame RAM Slicer/72 Bit Unpacker RAM 4/Unpack 72 Bit FIFO 1 ==
  72 Bit Input : Inport
  Slice 11 Down To 0 : hdlBasic/Slice  nbits=ScanlinePixelBitSizeController  boolean_output=off  mode=Upper Bit Location + Width  bit1=Slice11DownTo0Top  base1=LSB of Input  bit0=0  base0=Binary Point of Input  XmcBlockStatus=1  maskContainerNames=group1  block_type=slice  block_config=sysgen:Slice_config
  Slice 23 Down To 12 : hdlBasic/Slice  nbits=ScanlinePixelBitSizeController  boolean_output=off  mode=Upper Bit Location + Width  bit1=Slice23DownTo12Top  base1=LSB of Input  bit0=12  base0=Binary Point of Input  XmcBlockStatus=1  maskContainerNames=group1  block_type=slice  block_config=sysgen:Slice_config
  Slice 35 Down To 24 : hdlBasic/Slice  nbits=ScanlinePixelBitSizeController  boolean_output=off  mode=Upper Bit Location + Width  bit1=Slice35DownTo24Top  base1=LSB of Input  bit0=24  base0=Binary Point of Input  XmcBlockStatus=1  maskContainerNames=group1  block_type=slice  block_config=sysgen:Slice_config
  Slice 47 Down To 36 : hdlBasic/Slice  nbits=ScanlinePixelBitSizeController  boolean_output=off  mode=Upper Bit Location + Width  bit1=Slice47DownTo36Top  base1=LSB of Input  bit0=36  base0=Binary Point of Input  XmcBlockStatus=1  maskContainerNames=group1  block_type=slice  block_config=sysgen:Slice_config
  Slice 59 Down To 48 : hdlBasic/Slice  nbits=ScanlinePixelBitSizeController  boolean_output=off  mode=Upper Bit Location + Width  bit1=Slice59DownTo48Top  base1=LSB of Input  bit0=48  base0=Binary Point of Input  XmcBlockStatus=1  maskContainerNames=group1  block_type=slice  block_config=sysgen:Slice_config
  Slice 71 Down To 60 : hdlBasic/Slice  nbits=ScanlinePixelBitSizeController  boolean_output=off  mode=Upper Bit Location + Width  bit1=Slice71DownTo60Top  base1=LSB of Input  bit0=Slice71DownTo60Botttom  base0=LSB of Input  XmcBlockStatus=1  maskContainerNames=group1  block_type=slice  block_config=sysgen:Slice_config
  71 Downto 60 : Outport
  59 Downto 48 : Outport  Port=2
  47 Downto 36 : Outport  Port=3
  35 Downto 24 : Outport  Port=4
  23 Downto 12 : Outport  Port=5
  11 Downto 0 : Outport  Port=6
  wires:
  72 Bit Input/1 -> Slice 11 Down To 0/1, Slice 23 Down To 12/1, Slice 35 Down To 24/1, Slice 47 Down To 36/1, Slice 59 Down To 48/1, Slice 71 Down To 60/1
  Slice 23 Down To 12/1 -> 23 Downto 12/1
  Slice 47 Down To 36/1 -> 47 Downto 36/1
  Slice 59 Down To 48/1 -> 59 Downto 48/1
  Slice 35 Down To 24/1 -> 35 Downto 24/1
  Slice 71 Down To 60/1 -> 71 Downto 60/1
  Slice 11 Down To 0/1 -> 11 Downto 0/1

== system CMOS_Kernel_Memory_Sync/Memory Handler/Data Slicer/Kernel RAM Slicer/72 Bit Kernel Unpacker RAM 0/Unpack Kernel 72 Bit FIFO 0 ==
  72 Bit Input : Inport
  Slice 17 Down To 0 : hdlBasic/Slice  nbits=KernelWeightBitSizeController  boolean_output=off  mode=Upper Bit Location + Width  bit1=KernelSlice17DownTo0Top  base1=LSB of Input  bit0=0  base0=Binary Point of Input  XmcBlockStatus=1  maskContainerNames=group1  block_type=slice  block_config=sysgen:Slice_config
  Slice 35 Down To 18 : hdlBasic/Slice  nbits=KernelWeightBitSizeController  boolean_output=off  mode=Upper Bit Location + Width  bit1=KernelSlice35DownTo18Top  base1=LSB of Input  bit0=18  base0=Binary Point of Input  XmcBlockStatus=1  maskContainerNames=group1  block_type=slice  block_config=sysgen:Slice_config
  Slice 53 Down To 36 : hdlBasic/Slice  nbits=KernelWeightBitSizeController  boolean_output=off  mode=Upper Bit Location + Width  bit1=KernelSlice53DownTo36Top  base1=LSB of Input  bit0=36  base0=Binary Point of Input  XmcBlockStatus=1  maskContainerNames=group1  block_type=slice  block_config=sysgen:Slice_config
  Slice 71 Down To 54 : hdlBasic/Slice  nbits=KernelWeightBitSizeController  boolean_output=off  mode=Upper Bit Location + Width  bit1=KernelSlice71DownTo54Top  base1=LSB of Input  bit0=54  base0=Binary Point of Input  XmcBlockStatus=1  maskContainerNames=group1  block_type=slice  block_config=sysgen:Slice_config
  71 Downto 54 : Outport
  53 Downto 36 : Outport  Port=2
  35 Downto 18 : Outport  Port=3
  17 Downto 0 : Outport  Port=4
  wires:
  72 Bit Input/1 -> Slice 17 Down To 0/1, Slice 35 Down To 18/1, Slice 53 Down To 36/1, Slice 71 Down To 54/1
  Slice 35 Down To 18/1 -> 35 Downto 18/1
  Slice 53 Down To 36/1 -> 53 Downto 36/1
  Slice 17 Down To 0/1 -> 17 Downto 0/1
  Slice 71 Down To 54/1 -> 71 Downto 54/1

== system CMOS_Kernel_Memory_Sync/Memory Handler/Data Slicer/Kernel RAM Slicer/72 Bit Kernel Unpacker RAM 0/Unpack Kernel 72 Bit FIFO 1 ==
  72 Bit Input : Inport
  Slice 17 Down To 0 : hdlBasic/Slice  nbits=KernelWeightBitSizeController  boolean_output=off  mode=Upper Bit Location + Width  bit1=KernelSlice17DownTo0Top  base1=LSB of Input  bit0=0  base0=Binary Point of Input  XmcBlockStatus=1  maskContainerNames=group1  block_type=slice  block_config=sysgen:Slice_config
  Slice 35 Down To 18 : hdlBasic/Slice  nbits=KernelWeightBitSizeController  boolean_output=off  mode=Upper Bit Location + Width  bit1=KernelSlice35DownTo18Top  base1=LSB of Input  bit0=18  base0=Binary Point of Input  XmcBlockStatus=1  maskContainerNames=group1  block_type=slice  block_config=sysgen:Slice_config
  Slice 53 Down To 36 : hdlBasic/Slice  nbits=KernelWeightBitSizeController  boolean_output=off  mode=Upper Bit Location + Width  bit1=KernelSlice53DownTo36Top  base1=LSB of Input  bit0=36  base0=Binary Point of Input  XmcBlockStatus=1  maskContainerNames=group1  block_type=slice  block_config=sysgen:Slice_config
  Slice 71 Down To 54 : hdlBasic/Slice  nbits=KernelWeightBitSizeController  boolean_output=off  mode=Upper Bit Location + Width  bit1=KernelSlice71DownTo54Top  base1=LSB of Input  bit0=54  base0=Binary Point of Input  XmcBlockStatus=1  maskContainerNames=group1  block_type=slice  block_config=sysgen:Slice_config
  71 Downto 54 : Outport
  53 Downto 36 : Outport  Port=2
  35 Downto 18 : Outport  Port=3
  17 Downto 0 : Outport  Port=4
  wires:
  72 Bit Input/1 -> Slice 17 Down To 0/1, Slice 35 Down To 18/1, Slice 53 Down To 36/1, Slice 71 Down To 54/1
  Slice 35 Down To 18/1 -> 35 Downto 18/1
  Slice 53 Down To 36/1 -> 53 Downto 36/1
  Slice 17 Down To 0/1 -> 17 Downto 0/1
  Slice 71 Down To 54/1 -> 71 Downto 54/1

== system CMOS_Kernel_Memory_Sync/Memory Handler/Data Slicer/Kernel RAM Slicer/72 Bit Kernel Unpacker RAM 0/Unpack Kernel 72 Bit FIFO 2 ==
  72 Bit Input : Inport
  Slice 17 Down To 0 : hdlBasic/Slice  nbits=KernelWeightBitSizeController  boolean_output=off  mode=Upper Bit Location + Width  bit1=KernelSlice17DownTo0Top  base1=LSB of Input  bit0=0  base0=Binary Point of Input  XmcBlockStatus=1  maskContainerNames=group1  block_type=slice  block_config=sysgen:Slice_config
  Slice 35 Down To 18 : hdlBasic/Slice  nbits=KernelWeightBitSizeController  boolean_output=off  mode=Upper Bit Location + Width  bit1=KernelSlice35DownTo18Top  base1=LSB of Input  bit0=18  base0=Binary Point of Input  XmcBlockStatus=1  maskContainerNames=group1  block_type=slice  block_config=sysgen:Slice_config
  Slice 53 Down To 36 : hdlBasic/Slice  nbits=KernelWeightBitSizeController  boolean_output=off  mode=Upper Bit Location + Width  bit1=KernelSlice53DownTo36Top  base1=LSB of Input  bit0=36  base0=Binary Point of Input  XmcBlockStatus=1  maskContainerNames=group1  block_type=slice  block_config=sysgen:Slice_config
  Slice 71 Down To 54 : hdlBasic/Slice  nbits=KernelWeightBitSizeController  boolean_output=off  mode=Upper Bit Location + Width  bit1=KernelSlice71DownTo54Top  base1=LSB of Input  bit0=54  base0=Binary Point of Input  XmcBlockStatus=1  maskContainerNames=group1  block_type=slice  block_config=sysgen:Slice_config
  71 Downto 54 : Outport
  53 Downto 36 : Outport  Port=2
  35 Downto 18 : Outport  Port=3
  17 Downto 0 : Outport  Port=4
  wires:
  72 Bit Input/1 -> Slice 17 Down To 0/1, Slice 35 Down To 18/1, Slice 53 Down To 36/1, Slice 71 Down To 54/1
  Slice 35 Down To 18/1 -> 35 Downto 18/1
  Slice 53 Down To 36/1 -> 53 Downto 36/1
  Slice 17 Down To 0/1 -> 17 Downto 0/1
  Slice 71 Down To 54/1 -> 71 Downto 54/1
